simulink model "Exp4_PartB_19EE10039"  (R2021a)
settings: Solver=VariableStepAuto  StartTime=0.0  StopTime=0.04  RelTol=1e-3
libraries: spsThyristorLib x4, spsVoltageMeasurementLib x3, spsACVoltageSourceLib x2, spsGroundLib x2, spsMonostableLib x2, spspowerguiLib x2, spsSeriesRLCBranchLib x2, spsDiodeLib x1, spsDCVoltageSourceLib x1, simulink_extras x1, spsLinearTransformerLib x1
settings Model: Creator=USER  LastModifiedBy=mansi

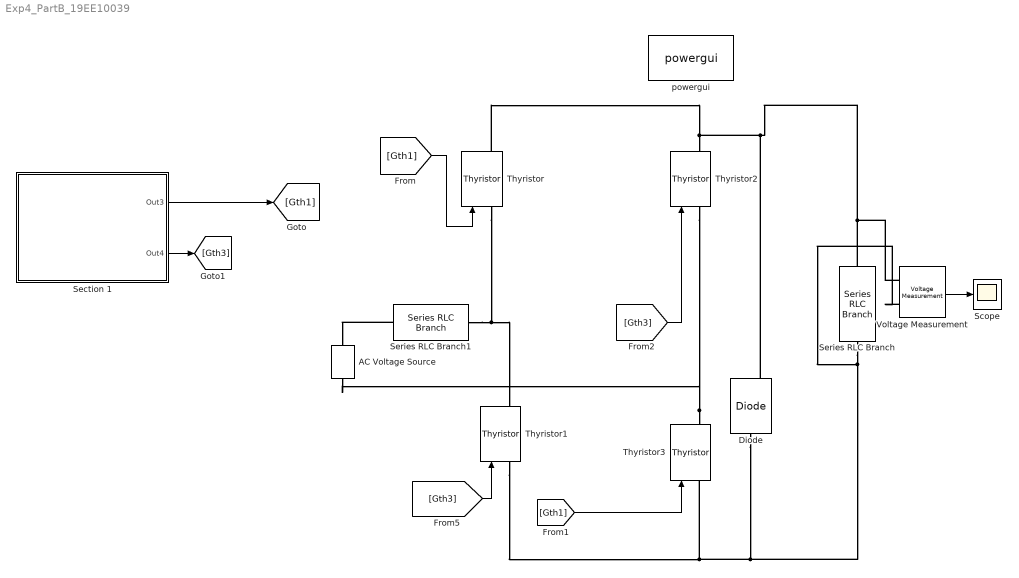
== system Exp4_PartB_19EE10039 ==
  AC Voltage Source : spsACVoltageSourceLib/AC Voltage Source  Amplitude=230*sqrt(2)  Phase=0  Frequency=50  SampleTime=0  Measurements=None  BusType=swing  Pref=10e3  Qref=0  Qmin=-inf  Qmax=+inf
  Diode : spsDiodeLib/Diode  Ron=1e-6  Lon=0  Vf=0  IC=0  UseSnubber=0  Rs=500  Cs=250e-9  Measurements=on
  Scope : Scope
  Section 1 : Subsystem
  Series RLC Branch : spsSeriesRLCBranchLib/Series RLC Branch  LConnTagsString=__new0  RConnTagsString=__new0  BranchType=RL  Resistance=22.416  Inductance=60e-3  SetiL0=off  InitialCurrent=0  Capacitance=1e-6  Setx0=off  InitialVoltage=0  Measurements=None
  Series RLC Branch1 : spsSeriesRLCBranchLib/Series RLC Branch  LConnTagsString=__new0  RConnTagsString=__new0  BranchType=L  Resistance=22.416  Inductance=2.5e-3  SetiL0=off  InitialCurrent=0  Capacitance=1e-6  Setx0=off  InitialVoltage=0  Measurements=None
  Thyristor{,1..3} (4 alike) : spsThyristorLib/Thyristor  Ron=1e-6  Lon=0  Vf=0  IC=0  Rs=500  Cs=250e-9  Measurements=on
  Voltage Measurement : spsVoltageMeasurementLib/Voltage Measurement  PhasorSimulation=off  OutputType=Complex  PSBequivalent=0
  powergui : spspowerguiLib/powergui  Priority=1  SimulationMode=Discrete  SampleTime=1e-6  frequency=60  Iterations=50  frequencyindice=0  Pbase=100e6  ErrMax=1e-4  UnitsV=kV  UnitsW=MW  buscounter=0  FunctionMessages=off  echomessages=off  EnableUseOfTLC=off  CurrentSourceSwitches=off  DisableSnubberDevices=off  DisableRonSwitches=off  DisableVfSwitches=off  DisplayEquations=off  AutomaticDiscreteSolvers=off  SolverType=Tustin/Backward Euler (TBE)  Interpol=off  ExternalGateDelay=off  methode=off  Ts=10  x0status=blocks  SPID=off  SwTol=0  HookPort=off  NonlinearTolerance=1e-4  nMaxIteration=100  ContinueOnMaxIteration=off  RestoreLinks=warning  ResistiveCurrentMeasurement=off  Frange=[0:2:500]  Ylog=off  Xlog=on  ShowGrid=off  save=off  variable=ZData  structure=ScopeData10  ZoomFFT=off  StartTime=0.124  cycles=2  DisplayStyle=2  fundamental=50  FreqAxis=on  MaxFrequency=5000  frequencyindicesteady=1  RmsSteady=1  display=off
  wires:
  [Gth1] -> Thyristor3/1
  [Gth3] -> Thyristor1/1
  [Gth3] -> Thyristor2/1
  [Gth1] -> Thyristor/1
  Voltage Measurement/1 -> Scope/1
  Section 1/1(Out3) -> [Gth1]
  Section 1/2(Out4) -> [Gth3]
  connections:
  Thyristor/LConn1 -- Series RLC Branch1/RConn1 -- Thyristor1/RConn1
  Voltage Measurement/LConn1 -- Series RLC Branch/RConn1 -- Diode/RConn1 -- Thyristor/RConn1 -- Thyristor2/RConn1
  Voltage Measurement/LConn2 -- Diode/LConn1 -- Thyristor1/LConn1 -- Thyristor3/LConn1 -- Series RLC Branch/LConn1
  Thyristor3/RConn1 -- AC Voltage Source/LConn1 -- Thyristor2/LConn1
  Series RLC Branch1/LConn1 -- AC Voltage Source/RConn1

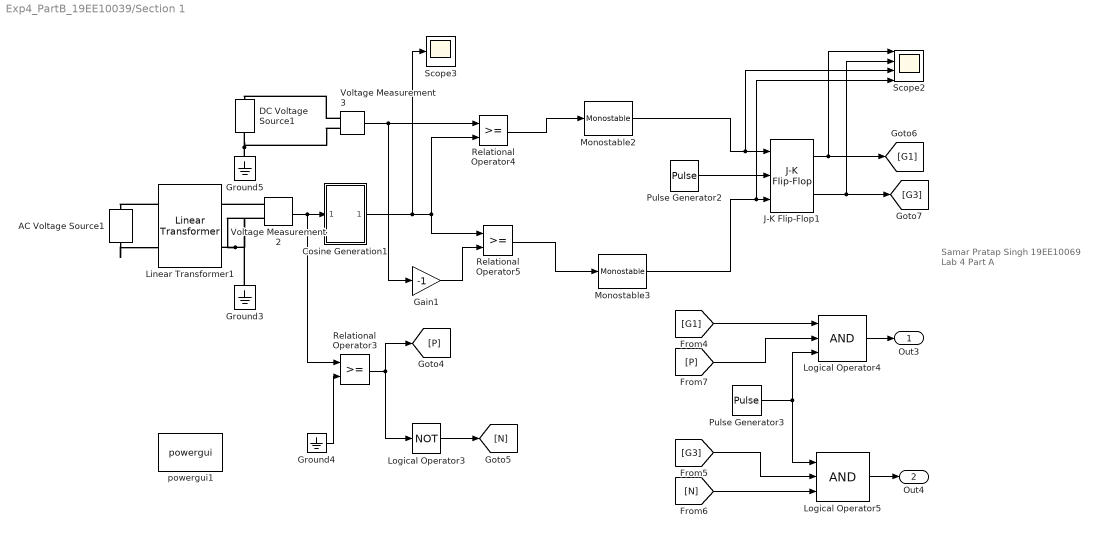
== system Exp4_PartB_19EE10039/Section 1 ==
  note: Samar Pratap Singh
      | 19EE10069
      | Lab 4
      | Part A
  AC Voltage Source1 : spsACVoltageSourceLib/AC Voltage Source  Amplitude=230*sqrt(2)  Phase=0  Frequency=50  SampleTime=0  Measurements=None  BusType=swing  Pref=10e3  Qref=0  Qmin=-inf  Qmax=+inf
  Cosine Generation1 : Subsystem
  DC Voltage Source1 : spsDCVoltageSourceLib/DC Voltage Source  Amplitude=4.015  Measurements=None
  Gain1 : Gain  Gain=-1
  Ground3 : spsGroundLib/Ground  LConnTagsString=a
  Ground4 : Ground
  Ground5 : spsGroundLib/Ground  LConnTagsString=a
  J-K Flip-Flop1 : simulink_extras/Flip Flops/J-K Flip-Flop  initial_condition=0
  Linear Transformer1 : spsLinearTransformerLib/Linear Transformer  UNITS=SI  NominalPower=[4 50]  winding1=[230 6.9 7.1e-3]  winding2=[3.605 1.7e-3 2.1e-6]  ThreeWindings=off  winding3=[3.15e+05 315.06 0.10641]  RmLm=[600 1.145]  Measurements=None  DataType=on
  Logical Operator3 : Logic  Operator=NOT  Inputs=1  IconShape=distinctive  AllPortsSameDT=off  OutDataTypeStr=boolean
  Logical Operator4 : Logic  Inputs=3  IconShape=distinctive  AllPortsSameDT=off  OutDataTypeStr=boolean
  Logical Operator5 : Logic  Inputs=3  IconShape=distinctive  AllPortsSameDT=off  OutDataTypeStr=boolean
  Monostable2 : spsMonostableLib/Monostable  EdgeDetect=Rising  PulseDuration=1e-5  ic=0  Ts=0
      settings: SourceProductBaseCode=PS
  Monostable3 : spsMonostableLib/Monostable  EdgeDetect=Rising  PulseDuration=1e-5  ic=0  Ts=0
      settings: SourceProductBaseCode=PS
  Pulse Generator2 : DiscretePulseGenerator  PulseType=Time based  Period=2e-6  PulseWidth=50
  Pulse Generator3 : DiscretePulseGenerator  PulseType=Time based  Period=40e-6  PulseWidth=50
  Relational Operator3 : RelationalOperator  OutDataTypeStr=boolean  RndMeth=Simplest
  Relational Operator4 : RelationalOperator  OutDataTypeStr=boolean  RndMeth=Simplest
  Relational Operator5 : RelationalOperator  OutDataTypeStr=boolean  RndMeth=Simplest
  Scope2 : Scope  NumInputPorts=4
  Scope3 : Scope
  Voltage Measurement2 : spsVoltageMeasurementLib/Voltage Measurement  PhasorSimulation=off  OutputType=Complex  PSBequivalent=0
  Voltage Measurement3 : spsVoltageMeasurementLib/Voltage Measurement  PhasorSimulation=off  OutputType=Complex  PSBequivalent=0
  powergui1 : spspowerguiLib/powergui  Priority=1  SimulationMode=Discrete  SampleTime=1e-6  frequency=60  Iterations=50  frequencyindice=0  Pbase=100e6  ErrMax=1e-4  UnitsV=kV  UnitsW=MW  buscounter=0  FunctionMessages=off  echomessages=off  EnableUseOfTLC=off  CurrentSourceSwitches=off  DisableSnubberDevices=off  DisableRonSwitches=off  DisableVfSwitches=off  DisplayEquations=off  AutomaticDiscreteSolvers=off  SolverType=Tustin/Backward Euler (TBE)  Interpol=off  ExternalGateDelay=off  methode=off  Ts=10  x0status=blocks  SPID=off  SwTol=0  HookPort=off  NonlinearTolerance=1e-4  nMaxIteration=100  ContinueOnMaxIteration=off  RestoreLinks=warning  ResistiveCurrentMeasurement=off  Frange=[0:2:500]  Ylog=off  Xlog=on  ShowGrid=off  save=off  variable=ZData  structure=ScopeData10  ZoomFFT=off  StartTime=0.124  cycles=2  DisplayStyle=2  fundamental=50  FreqAxis=on  MaxFrequency=5000  frequencyindicesteady=1  RmsSteady=1  display=off
  Out3 : Outport
  Out4 : Outport  Port=2
  wires:
  Relational Operator4/1 -> Monostable2/1
  Voltage Measurement3/1 -> Gain1/1, Relational Operator4/1
  Logical Operator3/1 -> [N]
  Voltage Measurement2/1 -> Cosine Generation1/1(In1), Relational Operator3/1
  [P] -> Logical Operator4/2
  J-K Flip-Flop1/2 -> Scope2/2, [G3]
  [G1] -> Logical Operator4/1
  Relational Operator3/1 -> [P], Logical Operator3/1
  Pulse Generator2/1 -> J-K Flip-Flop1/2
  [N] -> Logical Operator5/3
  Pulse Generator3/1 -> Logical Operator5/1, Logical Operator4/3
  Monostable2/1 -> Scope2/3, J-K Flip-Flop1/1
  Cosine Generation1/1(Out1) -> Scope3/1, Relational Operator4/2, Relational Operator5/1
  [G3] -> Logical Operator5/2
  Relational Operator5/1 -> Monostable3/1
  J-K Flip-Flop1/1 -> Scope2/1, [G1]
  Monostable3/1 -> Scope2/4, J-K Flip-Flop1/3
  Logical Operator5/1 -> Out4/1
  Gain1/1 -> Relational Operator5/2
  Ground4/1 -> Relational Operator3/2
  Logical Operator4/1 -> Out3/1
  connections:
  Linear Transformer1/RConn2 -- Voltage Measurement2/LConn2 -- Ground3/LConn1
  DC Voltage Source1/LConn1 -- Ground5/LConn1 -- Voltage Measurement3/LConn2
  Voltage Measurement2/LConn1 -- Linear Transformer1/RConn1
  AC Voltage Source1/LConn1 -- Linear Transformer1/LConn2
  Linear Transformer1/LConn1 -- AC Voltage Source1/RConn1
  Voltage Measurement3/LConn1 -- DC Voltage Source1/RConn1

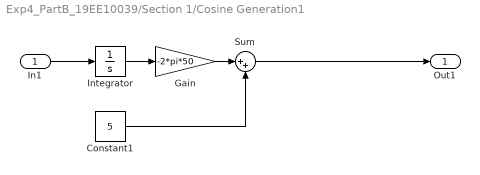
== system Exp4_PartB_19EE10039/Section 1/Cosine Generation1 ==
  In1 : Inport
  Constant1 : Constant  Value=5
  Gain : Gain  Gain=-2*pi*50
  Integrator : Integrator
  Sum : Sum  Inputs=|++
  Out1 : Outport
  wires:
  Sum/1 -> Out1/1
  Constant1/1 -> Sum/2
  In1/1 -> Integrator/1
  Integrator/1 -> Gain/1
  Gain/1 -> Sum/1
